simulink model "radia_team28_coilbuilder_dynamic"  (R2026a)
settings: Solver=FixedStepDiscrete  StopTime=2.0  FixedStep=team28_sample_time_s
model workspace (MAT data in the model file):
  radia_team28_coilbuilder_lut.schema = "radia.team28.lift_lut.v1"
  radia_team28_coilbuilder_lut.height_offset_m = [-0.007; -0.006; -0.005; -0.004; -0.003; -0.002; -0.001; 0; 0.001; 0.002; 0.003; 0.004; 0.005; 0.006; 0.007; 0.008; 0.009; 0.01; 0.011; 0.012; 0.013; 0.014; 0.015; 0.016; 0.017]
  radia_team28_coilbuilder_lut.force_N = [-3.31602873262; -2.85735084237; -2.45632234226; -2.10609263684; -1.80059648181; -1.5344663093; -1.30295460608; -1.10186468633; -0.927488851119; -0.776553169586; -0.646168226279; -0.533785243162; -0.437157035128; -0.354303302807; -0.283479809152; -0.223151027031; -0.171965883686; -0.128736264259; -0.0924179703173; -0.0620938605325; -0.036958929211; -0.0163071044041; 0.000480429079005; 0.0139455551353; 0.02456235453]
  radia_team28_coilbuilder_lut.upward_lift_N = [3.31602873262; 2.85735084237; 2.45632234226; 2.10609263684; 1.80059648181; 1.5344663093; 1.30295460608; 1.10186468633; 0.927488851119; 0.776553169586; 0.646168226279; 0.533785243162; 0.437157035128; 0.354303302807; 0.283479809152; 0.223151027031; 0.171965883686; 0.128736264259; 0.0924179703173; 0.0620938605325; 0.036958929211; 0.0163071044041; -0.000480429079005; -0.0139455551353; -0.02456235453]
  radia_team28_coilbuilder_lut.force_slope_N_per_m = [458.677890254; 429.853195182; 375.629102767; 327.862930226; 285.813163767; 248.820937865; 216.300811485; 187.732877479; 162.655758373; 140.66031242; 121.383963212; 104.505595576; 89.7409701776; 76.8386129877; 65.5761378881; 55.7569627332; 47.2073813858; 39.7739566844; 33.3212018633; 27.7295205531; 22.8933780642; 18.719679145; 15.1263297697; 12.0409627255; 10.6167993947]
  radia_team28_coilbuilder_lut.frequency_Hz = 50
  radia_team28_coilbuilder_lut.disk_weight_N = 1.055
  radia_team28_coilbuilder_lut.reference_coil_current_A = 20
  radia_team28_coilbuilder_lut.reference_disk_bottom_m = 0.0108
  radia_team28_coilbuilder_lut.physical_force_factor = 1
  radia_team28_coilbuilder_lut.sample_time_s = 0.001
  radia_team28_coilbuilder_lut.extrapolation = "clip"
  radia_team28_coilbuilder_lut.source_file = "validation_test\maglev\team28_coilbuilder_height_family_results.json"
  radia_team28_coilbuilder_lut.source_radia_version = "5.0.2"
  radia_team28_coilbuilder_lut.source_validation_passed = 1
  radia_team28_coilbuilder_lut.family_state_order = 3
  radia_team28_coilbuilder_lut.family_snapshot_count = 25
  radia_team28_coilbuilder_lut.coilbuilder_vector_potential_max_relative_l2 = 0.00061103999427
  radia_team28_coilbuilder_lut.coilbuilder_flux_density_max_relative_l2 = 0.00364217203549
  radia_team28_coilbuilder_lut.lift_curve_global_relative_error = 0.00816993731823
  radia_team28_coilbuilder_lut.equilibrium_offset_absolute_error_m = 2.93487831748e-05
  radia_team28_coilbuilder_lut.model = "TEAM 28 CoilBuilder + shared-mode Foster HCurl eddy-bubble height family"
  radia_team28_coilbuilder_lut.force_semantics = "fixed-frequency cycle-averaged Lorentz lift; current scales quadratically"
  team28_coil_current_A = 20
  team28_damping_Ns_per_m = 3.09121160251
  team28_disk_weight_N = 1.055
  team28_initial_height_offset_m = -0.007
  team28_inverse_mass_per_kg = 9.29857819905
  team28_reference_disk_bottom_m = 0.0108
  team28_sample_time_s = 0.001
undefined symbols (not defined in the file or in its folder): DiscIntNeverNeededParam
settings Model: Creator=Administrator  LastModifiedBy=Administrator

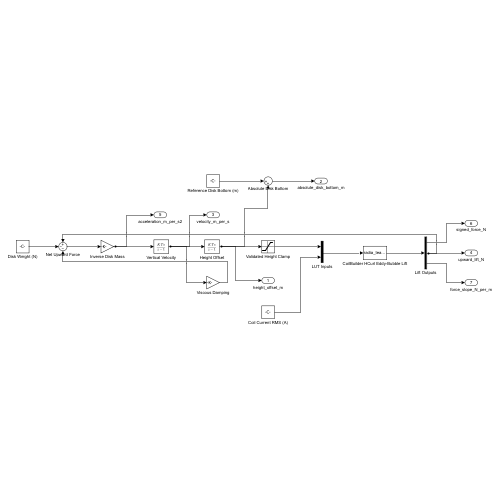
[thumbnail: Simulink's stored preview of the top-level diagram]
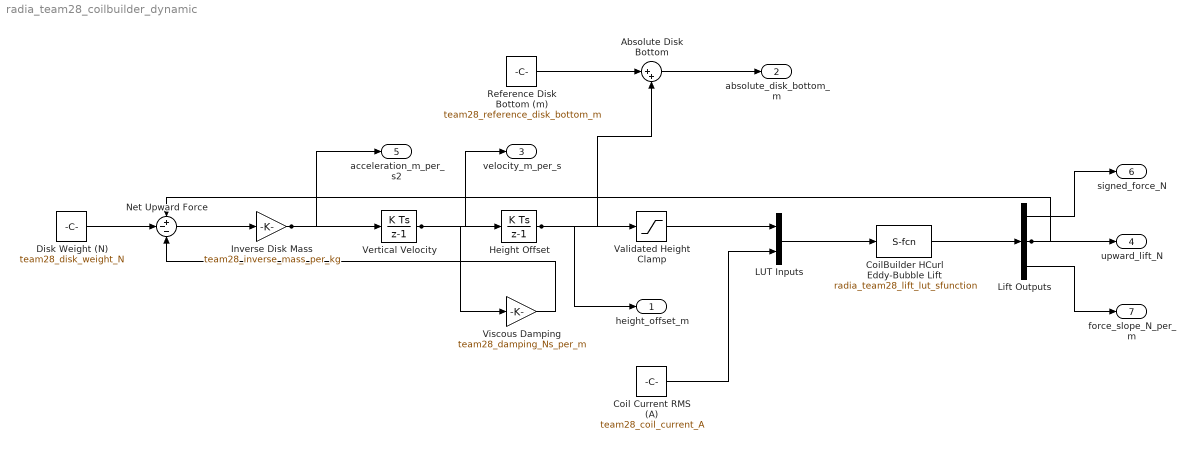
== system radia_team28_coilbuilder_dynamic ==
  Absolute Disk Bottom : Sum  Inputs=|++
  Coil Current RMS (A) : Constant  Value=team28_coil_current_A
  CoilBuilder HCurl Eddy-Bubble Lift : M-S-Function  FunctionName=radia_team28_lift_lut_sfunction  Parameters=radia_team28_coilbuilder_lut
  Disk Weight (N) : Constant  Value=team28_disk_weight_N
  Height Offset : DiscreteIntegrator  InitialCondition=team28_initial_height_offset_m  SampleTime=team28_sample_time_s  ICPrevOutput=DiscIntNeverNeededParam  ICPrevScaledInput=DiscIntNeverNeededParam
  Inverse Disk Mass : Gain  Gain=team28_inverse_mass_per_kg
  LUT Inputs : Mux  Inputs=2
  Lift Outputs : Demux  Outputs=3
  Net Upward Force : Sum  Inputs=+--
  Reference Disk Bottom (m) : Constant  Value=team28_reference_disk_bottom_m
  Validated Height Clamp : Saturate  UpperLimit=17e-3  LowerLimit=-7e-3
  Vertical Velocity : DiscreteIntegrator  SampleTime=team28_sample_time_s  ICPrevOutput=DiscIntNeverNeededParam  ICPrevScaledInput=DiscIntNeverNeededParam
  Viscous Damping : Gain  Gain=team28_damping_Ns_per_m
  height_offset_m : Outport
  absolute_disk_bottom_m : Outport  Port=2
  velocity_m_per_s : Outport  Port=3
  upward_lift_N : Outport  Port=4
  acceleration_m_per_s2 : Outport  Port=5
  signed_force_N : Outport  Port=6
  force_slope_N_per_m : Outport  Port=7
  wires:
  Lift Outputs/3 -> force_slope_N_per_m/1
  Lift Outputs/1 -> signed_force_N/1
  Absolute Disk Bottom/1 -> absolute_disk_bottom_m/1
  Reference Disk Bottom (m)/1 -> Absolute Disk Bottom/1
  Inverse Disk Mass/1 -> Vertical Velocity/1, acceleration_m_per_s2/1
  Net Upward Force/1 -> Inverse Disk Mass/1
  Viscous Damping/1 -> Net Upward Force/3
  Vertical Velocity/1 -> Viscous Damping/1, Height Offset/1, velocity_m_per_s/1
  Disk Weight (N)/1 -> Net Upward Force/2
  Lift Outputs/2 -> Net Upward Force/1, upward_lift_N/1
  Coil Current RMS (A)/1 -> LUT Inputs/2
  Validated Height Clamp/1 -> LUT Inputs/1
  Height Offset/1 -> Absolute Disk Bottom/2, Validated Height Clamp/1, height_offset_m/1
  LUT Inputs/1 -> CoilBuilder HCurl Eddy-Bubble Lift/1
  CoilBuilder HCurl Eddy-Bubble Lift/1 -> Lift Outputs/1
